simulink model "Hover"  (R2020a)
settings: Solver=ode3  StartTime=0.0  StopTime=20  FixedStep=0.001  RelTol=1e-3
model workspace (MAT data in the model file):
  C = 0.0001
  R = 1500
values from neighbouring files (symbols this model uses):
  T = 2.346    [Question3.m]
settings Model: OrderedModelArguments=off  Creator=shaun  LastModifiedBy=shaun

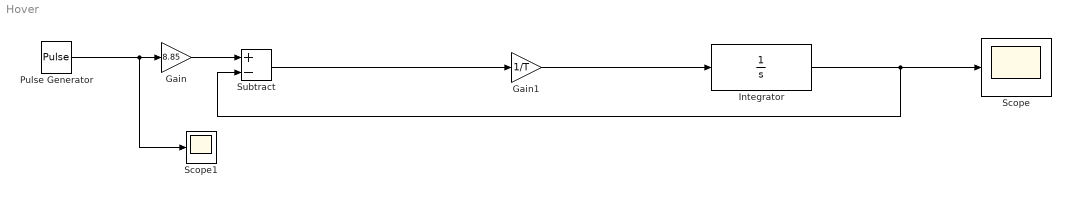
== system Hover ==
  Gain : Gain  Gain=8.85
  Gain1 : Gain  Gain=1/T
  Integrator : Integrator
  Pulse Generator : DiscretePulseGenerator  PulseType=Time based  Amplitude=1.508  Period=22  PulseWidth=50  PhaseDelay=1.5
  Scope : Scope
  Scope1 : Scope
  Subtract : Sum  Inputs=+-
  wires:
  Pulse Generator/1 -> Gain/1, Scope1/1
  Gain1/1 -> Integrator/1
  Subtract/1 -> Gain1/1
  Integrator/1 -> Subtract/2, Scope/1
  Gain/1 -> Subtract/1
